simulink model "untitled_4_71"  (Simulink 8.1)
settings: Solver=ode23tb  StartTime=0.0  StopTime=1  RelTol=1e-4
libraries: powerlib x11, powerlib_extras x8
settings Model: Creator=Nikola  LastModifiedBy=PC  BufferReuse=off
settings OptimizationCC: BlockReduction=off  InlineParams=on  BufferReuse=off

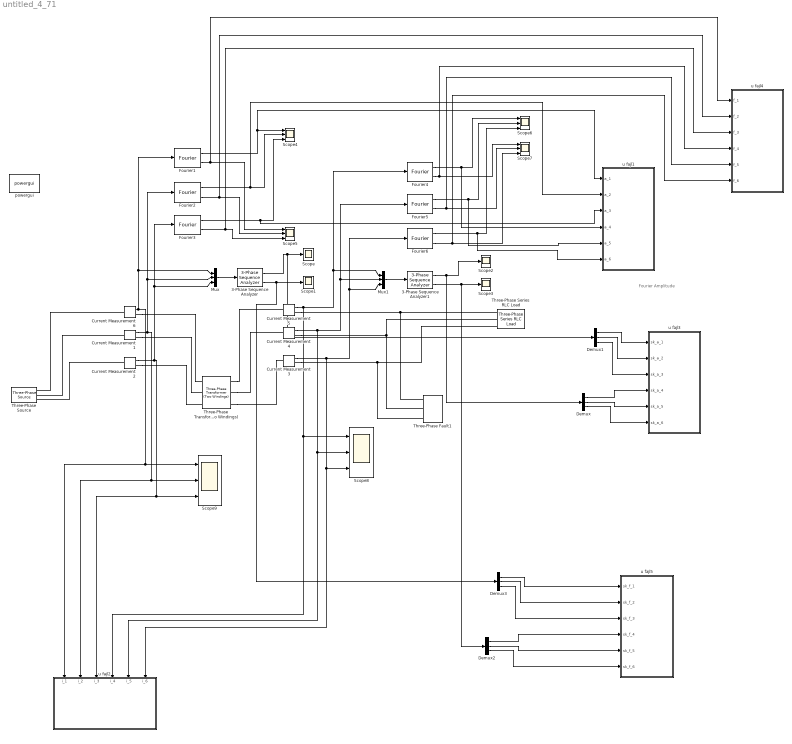
== system untitled_4_71 ==
  note: Fourier Amplitude
  3-Phase Sequence Analyzer : powerlib_extras/Measurements/3-Phase Sequence Analyzer  f1=50  n=1  seq=Positive Negative Zero
  3-Phase Sequence Analyzer1 : powerlib_extras/Measurements/3-Phase Sequence Analyzer  f1=50  n=1  seq=Positive Negative Zero
  Current Measurement{1..6} (6 alike) : powerlib/Measurements/Current Measurement  PhasorSimulation=off  OutputType=Complex  PSBequivalent=0
  Demux{,1..3} (4 alike) : Demux  Outputs=3
  Fourier{1..6} (6 alike) : powerlib_extras/Measurements/Fourier  f1=50  n=1
  Mux : Mux  Inputs=3
  Mux1 : Mux  Inputs=3
  Scope{,1..3} (4 alike) : Scope
      Scope settings: TimeRange=0.2  YMin=2.77556e-017  YMax=0.8
      Scope1 settings: TimeRange=0.2  YMin=-85  YMax=-80
      Scope2 settings: SaveName=ScopeData2
      Scope3 settings: SaveName=ScopeData3
  Scope{4..9} (6 alike) : Scope  NumInputPorts=3
      Scope4 settings: TimeRange=0.2  YMin=2.77556e-017~0~2.77556e-017  YMax=0.8~0.8~0.8  SaveName=ScopeData4
      Scope5 settings: TimeRange=0.2  YMin=-180~-180~35  YMax=180~180~40  SaveName=ScopeData5
      Scope6 settings: TimeRange=0.2  YMin=-5~-5~-5  YMax=5~5~5  SaveName=ScopeData6
      Scope7 settings: TimeRange=0.2  YMin=-5~-5~-5  YMax=5~5~5  SaveName=ScopeData7
      Scope8 settings: TimeRange=0.2  YMin=250~-120~10  YMax=2250~-40~120  SaveName=ScopeData8
      Scope9 settings: TimeRange=0.2  YMin=-180~-180~35  YMax=180~180~40  SaveName=ScopeData9
  Three-Phase Series RLC Load : powerlib/Elements/Three-Phase Series RLC Load  LConnTagsString=A|B|C  Configuration=Y (grounded)  NominalVoltage=6.3e3  NominalFrequency=50  ActivePower=0.9e6  InductivePower=0  CapacitivePower=0  Measurements=Branch currents  LoadType=constant PQ
  Three-Phase Transformer (Two Windings) : powerlib/Elements/Three-Phase Transformer (Two Windings)  Winding1Connection=Yg  UNITS=pu  NominalPower=[1e6 , 50 ]  Winding1=[20000 0.0017 0.05]  Winding2Connection=Yg  Winding2=[6300 0.0017 0.05]  SetSaturation=off  Rm=900  Lm=1600  Saturation=[0 0;0.30239 0.6;126 0.76001]  Hysteresis=off  DataFile='hysteresis'  SetInitialFlux=off  InitialFluxes=[-0.60398 0.66815 -0.064174]  Measurements=Winding currents  MoreParameters=off  BreakLoop=off  DataType=off  TransfoNumber=1
  Three-Phase Fault1 : powerlib/Elements/Three-Phase Fault  FaultA=on  FaultB=on  FaultC=on  FaultResistance=0.001  GroundFault=on  GroundResistance=0.001  External=off  SwitchStatus=[1]  SwitchTimes=[ 0.4 ]  InitialStates=[0 0 1]  SnubberResistance=1e6  SnubberCapacitance=inf  Measurements=Fault currents
  Three-Phase Source : powerlib/Electrical Sources/Three-Phase Source  Voltage=20e3  PhaseAngle=0  Frequency=50  InternalConnection=Yg  SpecifyImpedance=on  Resistance=0.8929  Inductance=16.58e-3  ShortCircuitLevel=500e6  BaseVoltage=20e3  XRratio=3.5  BusType=swing  Pref=0  Qref=0  Qmin=-inf  Qmax=inf
  powergui : powerlib/powergui  Priority=1  SimulationMode=Continuous  SolverType=Tustin  SampleTime=50e-6  frequency=60  SPID=off  DisableSnubberDevices=off  DisableRonSwitches=off  DisableVfSwitches=off  SwTol=0  Interpol=off  DisplayEquations=off  frequencyindice=0  Pbase=100e6  ErrMax=1e-4  Iterations=50  UnitsV=kV  UnitsW=MW  FunctionMessages=off  echomessages=off  HookPort=off  EnableUseOfTLC=off  x0status=blocks  RestoreLinks=warning  ResistiveCurrentMeasurement=off  Frange=[0:2:500]  Ylog=off  Xlog=on  ShowGrid=off  save=off  variable=ZData  ZoomFFT=off  StartTime=0.0  cycles=1  DisplayStyle=1  fundamental=60  FreqAxis=off  MaxFrequency=1000  frequencyindicesteady=1  RmsSteady=1  display=off  Ts=0  methode=off
  u fajl1 : Subsystem
  u fajl2 : Subsystem  StopFcn=graphs_loading_plots
  u fajl3 : Subsystem
  u fajl4 : Subsystem
  u fajl5 : Subsystem
  wires:
  Current Measurement6/1 -> Fourier1/1, Mux/1, Scope9/1, u fajl2/1(i_1)
  Current Measurement1/1 -> Fourier2/1, Mux/2, Scope9/2, u fajl2/2(i_2)
  Current Measurement2/1 -> Fourier3/1, Mux/3, Scope9/3, u fajl2/3(i_3)
  Mux/1 -> 3-Phase Sequence Analyzer/1
  3-Phase Sequence Analyzer/1 -> Scope/1, Demux1/1
  Current Measurement5/1 -> Fourier4/1, Mux1/1, u fajl2/4(i_4), Scope8/1
  Current Measurement4/1 -> Fourier5/1, Mux1/2, u fajl2/5(i_5), Scope8/2
  Current Measurement3/1 -> Fourier6/1, Mux1/3, u fajl2/6(i_6), Scope8/3
  Mux1/1 -> 3-Phase Sequence Analyzer1/1
  3-Phase Sequence Analyzer1/1 -> Scope2/1, Demux/1
  Fourier1/1 -> Scope4/1, u fajl1/1(a_1)
  Fourier2/1 -> Scope4/2, u fajl1/2(a_2)
  Fourier3/1 -> Scope4/3, u fajl1/3(a_3)
  Fourier1/2 -> Scope5/1, u fajl4/1(f_1)
  Fourier2/2 -> u fajl4/2(f_2), Scope5/2
  Fourier3/2 -> u fajl4/3(f_3), Scope5/3
  Fourier4/1 -> Scope6/1, u fajl1/4(a_4)
  Fourier5/1 -> Scope6/2, u fajl1/5(a_5)
  Fourier6/1 -> Scope6/3, u fajl1/6(a_6)
  Fourier4/2 -> Scope7/1, u fajl4/4(f_4)
  Fourier5/2 -> u fajl4/5(f_5), Scope7/2
  Fourier6/2 -> u fajl4/6(f_6), Scope7/3
  Demux/1 -> u fajl3/4(sk_a_4)
  Demux/2 -> u fajl3/5(sk_a_5)
  Demux/3 -> u fajl3/6(sk_a_6)
  Demux1/1 -> u fajl3/1(sk_a_1)
  Demux1/2 -> u fajl3/2(sk_a_2)
  Demux1/3 -> u fajl3/3(sk_a_3)
  3-Phase Sequence Analyzer/2 -> Demux3/1, Scope1/1
  3-Phase Sequence Analyzer1/2 -> Demux2/1, Scope3/1
  Demux2/1 -> u fajl5/4(sk_f_4)
  Demux2/2 -> u fajl5/5(sk_f_5)
  Demux2/3 -> u fajl5/6(sk_f_6)
  Demux3/1 -> u fajl5/1(sk_f_1)
  Demux3/2 -> u fajl5/2(sk_f_2)
  Demux3/3 -> u fajl5/3(sk_f_3)
  connections:
  Current Measurement6/LConn1 -- Three-Phase Source/RConn1
  Current Measurement1/LConn1 -- Three-Phase Source/RConn2
  Current Measurement2/RConn1 -- Three-Phase Transformer (Two Windings)/LConn3
  Current Measurement1/RConn1 -- Three-Phase Transformer (Two Windings)/LConn2
  Current Measurement6/RConn1 -- Three-Phase Transformer (Two Windings)/LConn1
  Three-Phase Transformer (Two Windings)/RConn1 -- Current Measurement5/LConn1
  Three-Phase Transformer (Two Windings)/RConn2 -- Current Measurement4/LConn1
  Three-Phase Transformer (Two Windings)/RConn3 -- Current Measurement3/LConn1
  Current Measurement4/RConn1 -- Three-Phase Series RLC Load/LConn2 -- Three-Phase Fault1/LConn2
  Three-Phase Fault1/LConn1 -- Current Measurement5/RConn1 -- Three-Phase Series RLC Load/LConn1
  Current Measurement3/RConn1 -- Three-Phase Series RLC Load/LConn3 -- Three-Phase Fault1/LConn3
  Current Measurement2/LConn1 -- Three-Phase Source/RConn3

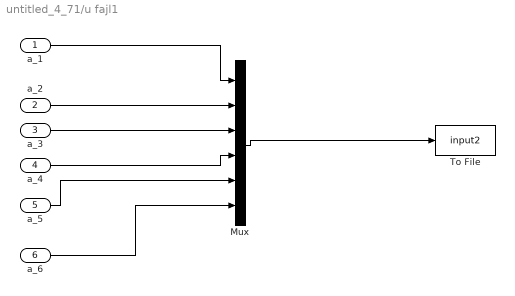
== system untitled_4_71/u fajl1 ==
  a_1 : Inport
  a_2 : Inport  Port=2
  a_3 : Inport  Port=3
  a_4 : Inport  Port=4
  a_5 : Inport  Port=5
  a_6 : Inport  Port=6
  Mux : Mux  Inputs=6
  To File : ToFile  Filename=input2  MatrixName=M2  SampleTime=0.02/100
  wires:
  Mux/1 -> To File/1
  a_1/1 -> Mux/1
  a_3/1 -> Mux/3
  a_4/1 -> Mux/4
  a_5/1 -> Mux/5
  a_6/1 -> Mux/6
  a_2/1 -> Mux/2

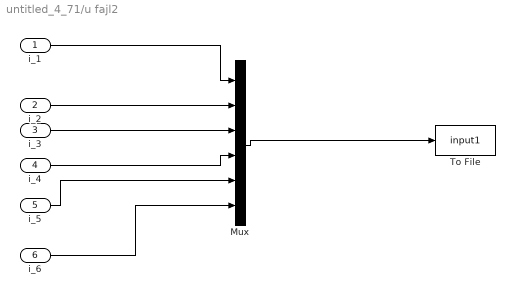
== system untitled_4_71/u fajl2 ==
  i_1 : Inport
  i_2 : Inport  Port=2
  i_3 : Inport  Port=3
  i_4 : Inport  Port=4
  i_5 : Inport  Port=5
  i_6 : Inport  Port=6
  Mux : Mux  Inputs=6
  To File : ToFile  Filename=input1  MatrixName=M  SampleTime=0.02/100
  wires:
  Mux/1 -> To File/1
  i_1/1 -> Mux/1
  i_3/1 -> Mux/3
  i_4/1 -> Mux/4
  i_5/1 -> Mux/5
  i_6/1 -> Mux/6
  i_2/1 -> Mux/2

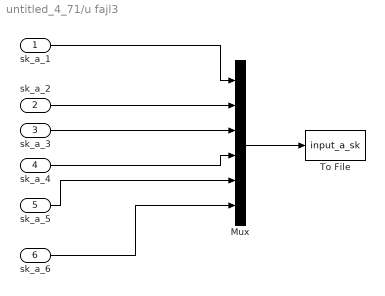
== system untitled_4_71/u fajl3 ==
  sk_a_1 : Inport
  sk_a_2 : Inport  Port=2
  sk_a_3 : Inport  Port=3
  sk_a_4 : Inport  Port=4
  sk_a_5 : Inport  Port=5
  sk_a_6 : Inport  Port=6
  Mux : Mux  Inputs=6
  To File : ToFile  Filename=input_a_sk  MatrixName=M_a_sk  SampleTime=0.02/100
  wires:
  Mux/1 -> To File/1
  sk_a_1/1 -> Mux/1
  sk_a_3/1 -> Mux/3
  sk_a_4/1 -> Mux/4
  sk_a_5/1 -> Mux/5
  sk_a_6/1 -> Mux/6
  sk_a_2/1 -> Mux/2

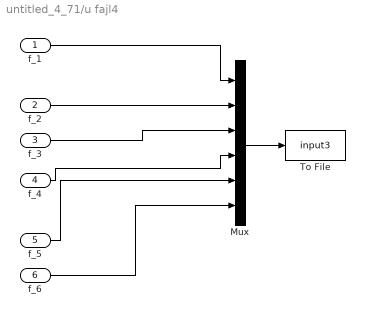
== system untitled_4_71/u fajl4 ==
  f_1 : Inport
  f_2 : Inport  Port=2
  f_3 : Inport  Port=3
  f_4 : Inport  Port=4
  f_5 : Inport  Port=5
  f_6 : Inport  Port=6
  Mux : Mux  Inputs=6
  To File : ToFile  Filename=input3  MatrixName=M3  SampleTime=0.02/100
  wires:
  Mux/1 -> To File/1
  f_1/1 -> Mux/1
  f_3/1 -> Mux/3
  f_4/1 -> Mux/4
  f_5/1 -> Mux/5
  f_6/1 -> Mux/6
  f_2/1 -> Mux/2

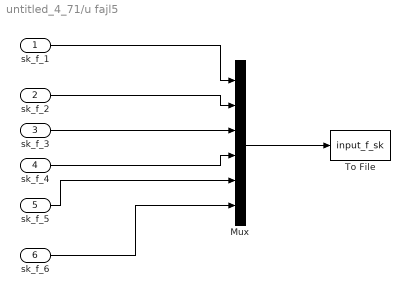
== system untitled_4_71/u fajl5 ==
  sk_f_1 : Inport
  sk_f_2 : Inport  Port=2
  sk_f_3 : Inport  Port=3
  sk_f_4 : Inport  Port=4
  sk_f_5 : Inport  Port=5
  sk_f_6 : Inport  Port=6
  Mux : Mux  Inputs=6
  To File : ToFile  Filename=input_f_sk  MatrixName=M_f_sk  SampleTime=0.02/100
  wires:
  Mux/1 -> To File/1
  sk_f_1/1 -> Mux/1
  sk_f_3/1 -> Mux/3
  sk_f_4/1 -> Mux/4
  sk_f_5/1 -> Mux/5
  sk_f_6/1 -> Mux/6
  sk_f_2/1 -> Mux/2
